simulink model "eng_model"  (R2023a)
settings: Solver=VariableStepAuto  StartTime=0.0  StopTime=30  RelTol=1e-3
undefined symbols (not defined in the file): C_m, C_w, J_eng, L_ov, L_ya, R_ya
settings Model: Creator=roma  LastModifiedBy=roma

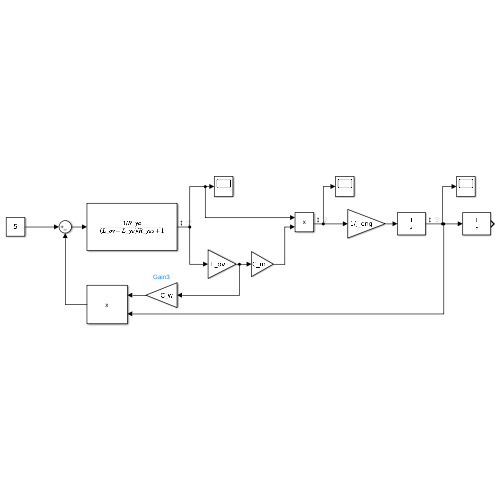
[thumbnail: Simulink's stored preview of the top-level diagram]
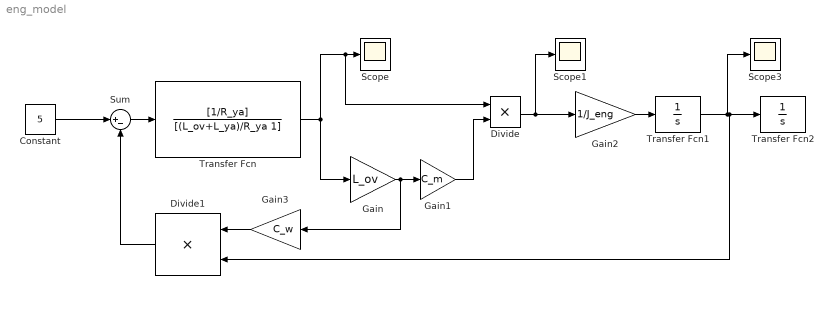
== system eng_model ==
  Constant : Constant  Value=5
  Divide : Product  Inputs=**
  Divide1 : Product  Inputs=**
  Gain : Gain  Gain=L_ov
  Gain1 : Gain  Gain=C_m
  Gain2 : Gain  Gain=1/J_eng
  Gain3 : Gain  Gain=C_w
  Scope : Scope
  Scope1 : Scope
  Scope3 : Scope
  Sum : Sum  Inputs=|+-
  Transfer Fcn : TransferFcn  Numerator=[1/R_ya]  Denominator=[(L_ov+L_ya)/R_ya 1]
  Transfer Fcn1 : TransferFcn  Denominator=[1 0]
  Transfer Fcn2 : TransferFcn  Denominator=[1 0]
  wires:
  Sum/1 -> Transfer Fcn/1
  Transfer Fcn/1 -> Gain/1, Divide/1, Scope/1
  Gain/1 -> Gain3/1, Gain1/1
  Gain1/1 -> Divide/2
  Divide/1 -> Scope1/1, Gain2/1
  Gain2/1 -> Transfer Fcn1/1
  Transfer Fcn1/1 -> Scope3/1, Transfer Fcn2/1, Divide1/2
  Gain3/1 -> Divide1/1
  Divide1/1 -> Sum/2
  Constant/1 -> Sum/1
